simulink subsystem "StewartPlatformInverseKinematics"  (R2022b)
settings: Solver=VariableStepAuto  StartTime=0.0  StopTime=10.0  RelTol=1e-3
settings Model: Creator=peter  LastModifiedBy=peter

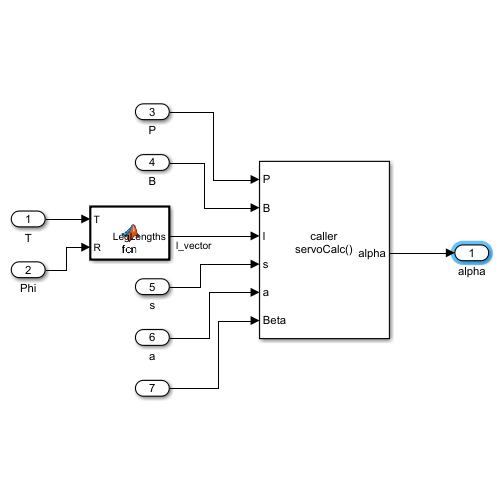
[thumbnail: Simulink's stored preview of the top-level diagram]
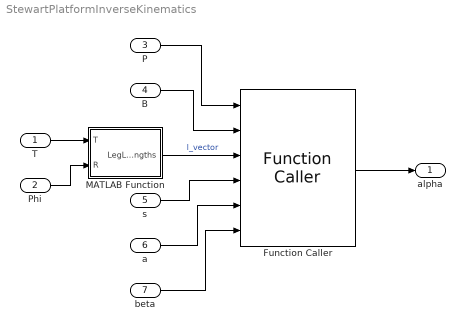
== system StewartPlatformInverseKinematics ==
  T : Inport
  Phi : Inport  Port=2
  P : Inport  Port=3
  B : Inport  Port=4
  s : Inport  Port=5
  a : Inport  Port=6
  beta : Inport  Port=7
  Function Caller : FunctionCaller  FunctionPrototype=alpha = servoCalc(P,B,l,s,a,beta)  InputArgumentSpecifications=<Enter example>  OutputArgumentSpecifications=<Enter example>
  MATLAB Function : MATLAB Function  TreatAsAtomicUnit=on
  alpha : Outport
  wires:
  T/1 -> MATLAB Function/1(T)
  beta/1 -> Function Caller/6
  a/1 -> Function Caller/5
  s/1 -> Function Caller/4
  Phi/1 -> MATLAB Function/2(R)
  MATLAB Function/1(LegLengths) -> Function Caller/3  "l_vector"
  B/1 -> Function Caller/2
  P/1 -> Function Caller/1
  Function Caller/1 -> alpha/1

== matlab function StewartPlatformInverseKinematics/MATLAB Function ==
  data: T input; LegLengths output; R input
function LegLengths = fcn(T, R)
LegLengths = (T + R*p) - b;
